simulink model "saturn_ib_stack"  (Simulink 6.2)
settings: Solver=ode4  SolverMode=SingleTasking  StartTime=0.0  StopTime=inf  FixedStep=0.005  RelTol=1e-3
values from neighbouring files (symbols this model uses):
  A_z_deg = 82.8200    (= 82.82)    [AS205_presettings.m]
  BN_1_sec = 14.4    [AS205_presettings.m]
  DeltaV_b_mps = 7.2381    [AS205_presettings.m]
  epsilon_2_sec = 15.0    (= 15)    [AS205_presettings.m]
  epsilon_prime_sec = 3.0    (= 3)    [AS205_presettings.m]
  i_deg = 28.89597    [AS205_presettings.m]
  lambda_0_deg = 102.32900    (= 102.329)    [AS205_presettings.m]
  lambda_L_deg = -80.561141    [AS205_presettings.m]
  pad_roll_L_deg = 100.0    (= 100)    [AS205_presettings.m]
  phi_L_deg = 28.521963    [AS205_presettings.m]
  phi_L_prime_deg = 28.360795    [AS205_presettings.m]
  R_L_m = 6373385.0    (= 6373385)    [AS205_presettings.m]
  R_T_m = 6570774.0    (= 6570774)    [AS205_presettings.m]
  T3_FM_sec = 6.08    [AS205_presettings.m]
  T_HSL_sec = 5.0    (= 5)    [AS205_presettings.m]
  Theta_T_deg = 0.000    (= 0)    [AS205_presettings.m]
  V_T_mps = 7780.976    [AS205_presettings.m]
  Xdotdot_VGT_mps2 = -9.251    [AS205_presettings.m]
undefined symbols (not defined in the file or in its folder): e0_0, e1_0, e2_0, e3_0, m, s
libraries: simulink x98, aerolibconvert x83, aerolibutil x63, aerolibtransform2 x34, aerolibasang x2, aerolibatmos2 x2, aerolib6dofsys x2
(part 6 of 7)

== system saturn_ib_stack/Saturn_IB_Stack/Saturn Instrument Unit (IU)/LVDA / LVDC/T4 Timer ==
  bStart : Inport  Port=1  DataType=boolean  LatchInput=off
  Clock : Clock
      settings: Decimation=10
  Constant : Constant  Value=0.0
  Data Store Memory : DataStoreMemory  DataStoreName=A  InitialValue=-1  DataType=double
  Data Store Read : DataStoreRead  DataStoreName=A  SampleTime=0
  Sum : Sum  Inputs=|+-
  Switch : Switch  Threshold=0.0
  Timer Initialization : Subsystem  TreatAsAtomicUnit=on
  T_elapsed_sec : Outport
  wires:
  bStart/1 -> Timer Initialization/Trigger
  Clock/1 -> Timer Initialization/1(In1), Sum/1
  Switch/1 -> T_elapsed_sec/1
  Sum/1 -> Switch/1
  Data Store Read/1 -> Sum/2, Switch/2
  Constant/1 -> Switch/3

== system saturn_ib_stack/Saturn_IB_Stack/Saturn Instrument Unit (IU)/ST-124M Stabilized Platform/Platform Gimbal Angles ==
  DCM : Inport  Port=1  LatchInput=off
  -sin(theta_x)cos(theta_z) : Fcn  Expr=-u(8)
  -sin(theta_y)cos(theta_z) : Fcn  Expr=-u(3)
  Mux2 : Mux  Inputs=3
  "Reshape 3x3 -> 9x1" : simulink/Math Operations/Reshape  OutputDimensionality=Customize  OutputDimensions=[9, 1]
  Trigonometric Function1 : Trigonometry  Operator=atan2
  Trigonometric Function3 : Trigonometry  Operator=atan2
  Trigonometric Function4 : Trigonometry  Operator=asin
  cos(theta_x)cos(theta_z) : Fcn  Expr=u(5)
  cos(theta_y)cos(theta_z) : Fcn  Expr=u(1)
  "sin(theta_z) " : Fcn  Expr=u(2)
  ST-124 Gimbal : Outport  InitialOutput=0
  wires:
  DCM/1 -> "Reshape 3x3 -> 9x1"/1
  "Reshape 3x3 -> 9x1"/1 -> -sin(theta_x)cos(theta_z)/1, cos(theta_x)cos(theta_z)/1, -sin(theta_y)cos(theta_z)/1, cos(theta_y)cos(theta_z)/1, "sin(theta_z) "/1
  -sin(theta_x)cos(theta_z)/1 -> Trigonometric Function1/1
  cos(theta_x)cos(theta_z)/1 -> Trigonometric Function1/2
  -sin(theta_y)cos(theta_z)/1 -> Trigonometric Function3/1
  cos(theta_y)cos(theta_z)/1 -> Trigonometric Function3/2
  Mux2/1 -> ST-124 Gimbal/1
  "sin(theta_z) "/1 -> Trigonometric Function4/1
  Trigonometric Function4/1 -> Mux2/3  "theta_z"
  Trigonometric Function1/1 -> Mux2/1  "theta_x"
  Trigonometric Function3/1 -> Mux2/2  "theta_y"

== system saturn_ib_stack/Saturn_IB_Stack/Initial Conditions/MES Transform/MES Transform/E-Frame to s-Frame (MES matrix) ==
  note: u(1)  sin Az
      | u(2)  sin Phi_L
      | u(3)  sin Theta_E
      | u(4)  cos Az
      | u(5)  cos Phi_L
      | u(6)  cos Theta_E
  note: Eqn 2.3.10
  Az phi_L Theta_E : Inport  Port=1  LatchInput=off
  11 : Fcn  Expr=u(5)*u(6)
  12 : Fcn  Expr=u(5)*u(3)
  13 : Fcn  Expr=u(2)
  21 : Fcn  Expr=u(2)*u(1)*u(6)-u(4)*u(3)
  22 : Fcn  Expr=u(2)*u(1)*u(3)+u(4)*u(6)
  23 : Fcn  Expr=-u(5)*u(1)
  31 : Fcn  Expr=-u(2)*u(4)*u(6)-u(1)*u(3)
  32 : Fcn  Expr=-u(2)*u(4)*u(3)+u(1)*u(6)
  33 : Fcn  Expr=u(5)*u(4)
  Mux : Mux  Inputs=2
  Mux2 : Mux  Inputs=9
  Reshape 9x1->3x3 : simulink/Math Operations/Reshape  OutputDimensionality=Customize  OutputDimensions=[3,3]
  SinCos3 : aerolibutil/SinCos
  DCM : Outport  InitialOutput=0
  wires:
  33/1 -> Mux2/9
  22/1 -> Mux2/5
  11/1 -> Mux2/1
  Mux2/1 -> Reshape 9x1->3x3/1
  Reshape 9x1->3x3/1 -> DCM/1
  Mux/1 -> 22/1, 11/1, 21/1, 31/1, 12/1, 32/1, 13/1, 33/1, 23/1
  23/1 -> Mux2/8
  13/1 -> Mux2/7
  32/1 -> Mux2/6
  12/1 -> Mux2/4
  31/1 -> Mux2/3
  21/1 -> Mux2/2
  Az phi_L Theta_E/1 -> SinCos3/1
  SinCos3/1 -> Mux/1
  SinCos3/2 -> Mux/2

== system saturn_ib_stack/Saturn_IB_Stack/On Pad/Initial Conditions/L/V Inertial Orientation/E-Frame to s-Frame (MES matrix) ==
  note: u(1)  sin Az
      | u(2)  sin Phi_L
      | u(3)  sin Theta_E
      | u(4)  cos Az
      | u(5)  cos Phi_L
      | u(6)  cos Theta_E
  note: Eqn 2.3.10
  Az phi_L Theta_E : Inport  Port=1  LatchInput=off
  11 : Fcn  Expr=u(5)*u(6)
  12 : Fcn  Expr=u(5)*u(3)
  13 : Fcn  Expr=u(2)
  21 : Fcn  Expr=u(2)*u(1)*u(6)-u(4)*u(3)
  22 : Fcn  Expr=u(2)*u(1)*u(3)+u(4)*u(6)
  23 : Fcn  Expr=-u(5)*u(1)
  31 : Fcn  Expr=-u(2)*u(4)*u(6)-u(1)*u(3)
  32 : Fcn  Expr=-u(2)*u(4)*u(3)+u(1)*u(6)
  33 : Fcn  Expr=u(5)*u(4)
  Mux : Mux  Inputs=2
  Mux2 : Mux  Inputs=9
  Reshape 9x1->3x3 : simulink/Math Operations/Reshape  OutputDimensionality=Customize  OutputDimensions=[3,3]
  SinCos3 : aerolibutil/SinCos
  DCM : Outport  InitialOutput=0
  wires:
  33/1 -> Mux2/9
  22/1 -> Mux2/5
  11/1 -> Mux2/1
  Mux2/1 -> Reshape 9x1->3x3/1
  Reshape 9x1->3x3/1 -> DCM/1
  Mux/1 -> 22/1, 11/1, 21/1, 31/1, 12/1, 32/1, 13/1, 33/1, 23/1
  23/1 -> Mux2/8
  13/1 -> Mux2/7
  32/1 -> Mux2/6
  12/1 -> Mux2/4
  31/1 -> Mux2/3
  21/1 -> Mux2/2
  Az phi_L Theta_E/1 -> SinCos3/1
  SinCos3/1 -> Mux/1
  SinCos3/2 -> Mux/2

== system saturn_ib_stack/Saturn_IB_Stack/On Pad/Initial Conditions/MES Transform/MES Transform ==
  A_z_deg : Inport  Port=1  LatchInput=off
  phi_L_deg : Inport  Port=2  LatchInput=off
  Theta_E_deg : Inport  Port=3  LatchInput=off
  Angle Conversion2 : aerolibconvert/Angle Conversion  IU=deg  OU=rad
  E-Frame to s-Frame (MES matrix) : Subsystem  AncestorBlock="aerolibtransform2/Euler Angles to  Direction Cosine Matrix"
      mask Type: Euler2DCM
      mask Description: Determine the 3-by-3 direction cosine matrix (DCM) transforming the E-frame to the S-Frame
      mask Display: disp('MES')
  Mux : Mux  Inputs=3
  DCM : Outport
  wires:
  phi_L_deg/1 -> Mux/2
  Theta_E_deg/1 -> Mux/3
  A_z_deg/1 -> Mux/1
  Mux/1 -> Angle Conversion2/1
  E-Frame to s-Frame (MES matrix)/1(DCM) -> DCM/1
  Angle Conversion2/1 -> E-Frame to s-Frame (MES matrix)/1(Az phi_L Theta_E)

== system saturn_ib_stack/Saturn_IB_Stack/S-IB Stage/Custom Variable Mass 6DoF (Quaternion)/Calculate DCM & Euler Angles/qdot ==
  p q r : Inport  Port=1  LatchInput=off
  q0 q1 q2 q3 : Inport  Port=2  LatchInput=off
  Constant : Constant
  Dot Product : simulink/Math Operations/Dot Product  OutDataType=sfix(16)  OutScaling=2^-10  DoSatur=off
  High Gain Quaternion Normalization : Gain  Gain=k_quat  SaturateOnIntegerOverflow=on
  Mux1 : Mux  Inputs=[3 4 1]
  Mux2 : Mux
  Sum : Sum  Inputs=|+-  SaturateOnIntegerOverflow=on  InputSameDT=on
  q0dot : Fcn  Expr=-0.5 * ( u[5]*u[1]+u[6]*u[2]+u[7]*u[3] ) + u[8]*u[4]
  q1dot : Fcn  Expr=0.5 * ( u[4]*u[1]+u[6]*u[3]-u[7]*u[2] ) + u[8]*u[5]
  q2dot : Fcn  Expr=0.5 * ( u[4]*u[2]+u[7]*u[1]-u[5]*u[3] ) + u[8]*u[6]
  q3dot : Fcn  Expr=0.5 * ( u[4]*u[3]+u[5]*u[2]-u[6]*u[1] ) + u[8]*u[7]
  qdot : Outport  InitialOutput=0
  wires:
  p q r/1 -> Mux1/1
  Dot Product/1 -> Sum/2
  High Gain Quaternion Normalization/1 -> Mux1/3
  Sum/1 -> High Gain Quaternion Normalization/1
  Constant/1 -> Sum/1
  Mux2/1 -> qdot/1
  q0dot/1 -> Mux2/1
  q1dot/1 -> Mux2/2
  q2dot/1 -> Mux2/3
  Mux1/1 -> q2dot/1, q3dot/1, q0dot/1, q1dot/1
  q3dot/1 -> Mux2/4
  q0 q1 q2 q3/1 -> Dot Product/1, Dot Product/2, Mux1/2

== system saturn_ib_stack/Saturn_IB_Stack/S-IB Stage/Custom Variable Mass 6DoF (Quaternion)/Calculate omega_dot/I x w ==
  p q r : Inport  Port=1  LatchInput=off
  Inertia : Inport  Port=2  LatchInput=off
  Product : Product  Multiplication=Matrix(*)  SaturateOnIntegerOverflow=on  InputSameDT=on
  I * w : Outport
  wires:
  p q r/1 -> Product/2
  Inertia/1 -> Product/1
  Product/1 -> I * w/1

== system saturn_ib_stack/Saturn_IB_Stack/S-IB Stage/Custom Variable Mass 6DoF (Quaternion)/Calculate omega_dot/I x w1 ==
  I_dot : Inport  Port=1  LatchInput=off
  p q r : Inport  Port=2  LatchInput=off
  Product : Product  Multiplication=Matrix(*)  SaturateOnIntegerOverflow=on  InputSameDT=on
  Id * w : Outport
  wires:
  Product/1 -> Id * w/1
  I_dot/1 -> Product/1
  p q r/1 -> Product/2

== system saturn_ib_stack/Saturn_IB_Stack/S-IB Stage/H-1 Engine Cluster/Engine 1/Triggered Timer ==
  bStart : Inport  Port=1  DataType=boolean  LatchInput=off
  Clock : Clock
      settings: Decimation=10
  Constant : Constant  Value=0.0
  Data Store Memory : DataStoreMemory  DataStoreName=A  InitialValue=-1  DataType=double
  Data Store Read : DataStoreRead  DataStoreName=A  SampleTime=0
  Sum : Sum  Inputs=|+-
  Switch : Switch  Threshold=0.0
  Timer Initialization : Subsystem  TreatAsAtomicUnit=on
  T_elapsed_sec : Outport
  wires:
  bStart/1 -> Timer Initialization/Trigger
  Clock/1 -> Timer Initialization/1(In1), Sum/1
  Switch/1 -> T_elapsed_sec/1
  Sum/1 -> Switch/1
  Data Store Read/1 -> Sum/2, Switch/2
  Constant/1 -> Switch/3

== system saturn_ib_stack/Saturn_IB_Stack/S-IB Stage/H-1 Engine Cluster/Engine 2/Triggered Timer ==
  bStart : Inport  Port=1  DataType=boolean  LatchInput=off
  Clock : Clock
      settings: Decimation=10
  Constant : Constant  Value=0.0
  Data Store Memory : DataStoreMemory  DataStoreName=A  InitialValue=-1  DataType=double
  Data Store Read : DataStoreRead  DataStoreName=A  SampleTime=0
  Sum : Sum  Inputs=|+-
  Switch : Switch  Threshold=0.0
  Timer Initialization : Subsystem  TreatAsAtomicUnit=on
  T_elapsed_sec : Outport
  wires:
  bStart/1 -> Timer Initialization/Trigger
  Clock/1 -> Timer Initialization/1(In1), Sum/1
  Switch/1 -> T_elapsed_sec/1
  Sum/1 -> Switch/1
  Data Store Read/1 -> Sum/2, Switch/2
  Constant/1 -> Switch/3

== system saturn_ib_stack/Saturn_IB_Stack/S-IB Stage/H-1 Engine Cluster/Engine 3/Triggered Timer ==
  bStart : Inport  Port=1  DataType=boolean  LatchInput=off
  Clock : Clock
      settings: Decimation=10
  Constant : Constant  Value=0.0
  Data Store Memory : DataStoreMemory  DataStoreName=A  InitialValue=-1  DataType=double
  Data Store Read : DataStoreRead  DataStoreName=A  SampleTime=0
  Sum : Sum  Inputs=|+-
  Switch : Switch  Threshold=0.0
  Timer Initialization : Subsystem  TreatAsAtomicUnit=on
  T_elapsed_sec : Outport
  wires:
  bStart/1 -> Timer Initialization/Trigger
  Clock/1 -> Timer Initialization/1(In1), Sum/1
  Switch/1 -> T_elapsed_sec/1
  Sum/1 -> Switch/1
  Data Store Read/1 -> Sum/2, Switch/2
  Constant/1 -> Switch/3

== system saturn_ib_stack/Saturn_IB_Stack/S-IB Stage/H-1 Engine Cluster/Engine 4/Triggered Timer ==
  bStart : Inport  Port=1  DataType=boolean  LatchInput=off
  Clock : Clock
      settings: Decimation=10
  Constant : Constant  Value=0.0
  Data Store Memory : DataStoreMemory  DataStoreName=A  InitialValue=-1  DataType=double
  Data Store Read : DataStoreRead  DataStoreName=A  SampleTime=0
  Sum : Sum  Inputs=|+-
  Switch : Switch  Threshold=0.0
  Timer Initialization : Subsystem  TreatAsAtomicUnit=on
  T_elapsed_sec : Outport
  wires:
  bStart/1 -> Timer Initialization/Trigger
  Clock/1 -> Timer Initialization/1(In1), Sum/1
  Switch/1 -> T_elapsed_sec/1
  Sum/1 -> Switch/1
  Data Store Read/1 -> Sum/2, Switch/2
  Constant/1 -> Switch/3

== system saturn_ib_stack/Saturn_IB_Stack/S-IB Stage/H-1 Engine Cluster/Engine 5/Triggered Timer ==
  bStart : Inport  Port=1  DataType=boolean  LatchInput=off
  Clock : Clock
      settings: Decimation=10
  Constant : Constant  Value=0.0
  Data Store Memory : DataStoreMemory  DataStoreName=A  InitialValue=-1  DataType=double
  Data Store Read : DataStoreRead  DataStoreName=A  SampleTime=0
  Sum : Sum  Inputs=|+-
  Switch : Switch  Threshold=0.0
  Timer Initialization : Subsystem  TreatAsAtomicUnit=on
  T_elapsed_sec : Outport
  wires:
  bStart/1 -> Timer Initialization/Trigger
  Clock/1 -> Timer Initialization/1(In1), Sum/1
  Switch/1 -> T_elapsed_sec/1
  Sum/1 -> Switch/1
  Data Store Read/1 -> Sum/2, Switch/2
  Constant/1 -> Switch/3

== system saturn_ib_stack/Saturn_IB_Stack/S-IB Stage/H-1 Engine Cluster/Engine 6/Triggered Timer ==
  bStart : Inport  Port=1  DataType=boolean  LatchInput=off
  Clock : Clock
      settings: Decimation=10
  Constant : Constant  Value=0.0
  Data Store Memory : DataStoreMemory  DataStoreName=A  InitialValue=-1  DataType=double
  Data Store Read : DataStoreRead  DataStoreName=A  SampleTime=0
  Sum : Sum  Inputs=|+-
  Switch : Switch  Threshold=0.0
  Timer Initialization : Subsystem  TreatAsAtomicUnit=on
  T_elapsed_sec : Outport
  wires:
  bStart/1 -> Timer Initialization/Trigger
  Clock/1 -> Timer Initialization/1(In1), Sum/1
  Switch/1 -> T_elapsed_sec/1
  Sum/1 -> Switch/1
  Data Store Read/1 -> Sum/2, Switch/2
  Constant/1 -> Switch/3

== system saturn_ib_stack/Saturn_IB_Stack/S-IB Stage/H-1 Engine Cluster/Engine 7/Triggered Timer ==
  bStart : Inport  Port=1  DataType=boolean  LatchInput=off
  Clock : Clock
      settings: Decimation=10
  Constant : Constant  Value=0.0
  Data Store Memory : DataStoreMemory  DataStoreName=A  InitialValue=-1  DataType=double
  Data Store Read : DataStoreRead  DataStoreName=A  SampleTime=0
  Sum : Sum  Inputs=|+-
  Switch : Switch  Threshold=0.0
  Timer Initialization : Subsystem  TreatAsAtomicUnit=on
  T_elapsed_sec : Outport
  wires:
  bStart/1 -> Timer Initialization/Trigger
  Clock/1 -> Timer Initialization/1(In1), Sum/1
  Switch/1 -> T_elapsed_sec/1
  Sum/1 -> Switch/1
  Data Store Read/1 -> Sum/2, Switch/2
  Constant/1 -> Switch/3

== system saturn_ib_stack/Saturn_IB_Stack/S-IB Stage/H-1 Engine Cluster/Engine 8/Triggered Timer ==
  bStart : Inport  Port=1  DataType=boolean  LatchInput=off
  Clock : Clock
      settings: Decimation=10
  Constant : Constant  Value=0.0
  Data Store Memory : DataStoreMemory  DataStoreName=A  InitialValue=-1  DataType=double
  Data Store Read : DataStoreRead  DataStoreName=A  SampleTime=0
  Sum : Sum  Inputs=|+-
  Switch : Switch  Threshold=0.0
  Timer Initialization : Subsystem  TreatAsAtomicUnit=on
  T_elapsed_sec : Outport
  wires:
  bStart/1 -> Timer Initialization/Trigger
  Clock/1 -> Timer Initialization/1(In1), Sum/1
  Switch/1 -> T_elapsed_sec/1
  Sum/1 -> Switch/1
  Data Store Read/1 -> Sum/2, Switch/2
  Constant/1 -> Switch/3

== system saturn_ib_stack/Saturn_IB_Stack/S-IB Stage/Retrorocket Motors/Time Since Engine Start/Timer Initialization ==
  In1 : Inport  Port=1  LatchInput=off
  Trigger : TriggerPort
  Data Store Write : DataStoreWrite  DataStoreName=A  SampleTime=-1
  wires:
  In1/1 -> Data Store Write/1

== system saturn_ib_stack/Saturn_IB_Stack/S-IVB Stage/Custom Variable Mass 6DoF (Quaternion)/Calculate DCM & Euler Angles/qdot ==
  p q r : Inport  Port=1  LatchInput=off
  q0 q1 q2 q3 : Inport  Port=2  LatchInput=off
  Constant : Constant
  Dot Product : simulink/Math Operations/Dot Product  OutDataType=sfix(16)  OutScaling=2^-10  DoSatur=off
  High Gain Quaternion Normalization : Gain  Gain=k_quat  SaturateOnIntegerOverflow=on
  Mux1 : Mux  Inputs=[3 4 1]
  Mux2 : Mux
  Sum : Sum  Inputs=|+-  SaturateOnIntegerOverflow=on  InputSameDT=on
  q0dot : Fcn  Expr=-0.5 * ( u[5]*u[1]+u[6]*u[2]+u[7]*u[3] ) + u[8]*u[4]
  q1dot : Fcn  Expr=0.5 * ( u[4]*u[1]+u[6]*u[3]-u[7]*u[2] ) + u[8]*u[5]
  q2dot : Fcn  Expr=0.5 * ( u[4]*u[2]+u[7]*u[1]-u[5]*u[3] ) + u[8]*u[6]
  q3dot : Fcn  Expr=0.5 * ( u[4]*u[3]+u[5]*u[2]-u[6]*u[1] ) + u[8]*u[7]
  qdot : Outport  InitialOutput=0
  wires:
  p q r/1 -> Mux1/1
  Dot Product/1 -> Sum/2
  High Gain Quaternion Normalization/1 -> Mux1/3
  Sum/1 -> High Gain Quaternion Normalization/1
  Constant/1 -> Sum/1
  Mux2/1 -> qdot/1
  q0dot/1 -> Mux2/1
  q1dot/1 -> Mux2/2
  q2dot/1 -> Mux2/3
  Mux1/1 -> q2dot/1, q3dot/1, q0dot/1, q1dot/1
  q3dot/1 -> Mux2/4
  q0 q1 q2 q3/1 -> Dot Product/1, Dot Product/2, Mux1/2

== system saturn_ib_stack/Saturn_IB_Stack/S-IVB Stage/Custom Variable Mass 6DoF (Quaternion)/Calculate omega_dot/I x w ==
  p q r : Inport  Port=1  LatchInput=off
  Inertia : Inport  Port=2  LatchInput=off
  Product : Product  Multiplication=Matrix(*)  SaturateOnIntegerOverflow=on  InputSameDT=on
  I * w : Outport
  wires:
  p q r/1 -> Product/2
  Inertia/1 -> Product/1
  Product/1 -> I * w/1

== system saturn_ib_stack/Saturn_IB_Stack/S-IVB Stage/Custom Variable Mass 6DoF (Quaternion)/Calculate omega_dot/I x w1 ==
  I_dot : Inport  Port=1  LatchInput=off
  p q r : Inport  Port=2  LatchInput=off
  Product : Product  Multiplication=Matrix(*)  SaturateOnIntegerOverflow=on  InputSameDT=on
  Id * w : Outport
  wires:
  Product/1 -> Id * w/1
  I_dot/1 -> Product/1
  p q r/1 -> Product/2

== system saturn_ib_stack/Saturn_IB_Stack/S-IVB Stage/J-2 Engine/Thrust Model/Time Since Engine Start ==
  bStart : Inport  Port=1  DataType=boolean  LatchInput=off
  Clock : Clock
      settings: Decimation=10
  Constant : Constant  Value=0.0
  Data Store Memory : DataStoreMemory  DataStoreName=A  InitialValue=-1  DataType=double
  Data Store Read : DataStoreRead  DataStoreName=A  SampleTime=0
  Sum : Sum  Inputs=|+-
  Switch : Switch  Threshold=0.0
  Timer Initialization : Subsystem  TreatAsAtomicUnit=on
  T_elapsed_sec : Outport
  wires:
  bStart/1 -> Timer Initialization/Trigger
  Clock/1 -> Timer Initialization/1(In1), Sum/1
  Switch/1 -> T_elapsed_sec/1
  Sum/1 -> Switch/1
  Data Store Read/1 -> Sum/2, Switch/2
  Constant/1 -> Switch/3

== system saturn_ib_stack/Saturn_IB_Stack/S-IVB Stage/J-2 Engine/Thrust Model/Time Since Shutdown ==
  bStart : Inport  Port=1  DataType=boolean  LatchInput=off
  Clock : Clock
      settings: Decimation=10
  Constant : Constant  Value=0.0
  Data Store Memory : DataStoreMemory  DataStoreName=A  InitialValue=-1  DataType=double
  Data Store Read : DataStoreRead  DataStoreName=A  SampleTime=0
  Sum : Sum  Inputs=|+-
  Switch : Switch  Threshold=0.0
  Timer Initialization : Subsystem  TreatAsAtomicUnit=on
  T_elapsed_sec : Outport
  wires:
  bStart/1 -> Timer Initialization/Trigger
  Clock/1 -> Timer Initialization/1(In1), Sum/1
  Switch/1 -> T_elapsed_sec/1
  Sum/1 -> Switch/1
  Data Store Read/1 -> Sum/2, Switch/2
  Constant/1 -> Switch/3

== system saturn_ib_stack/Saturn_IB_Stack/S-IVB Stage/Ullage Rocket Motors/Time Since Engine Start/Timer Initialization ==
  In1 : Inport  Port=1  LatchInput=off
  Trigger : TriggerPort
  Data Store Write : DataStoreWrite  DataStoreName=A  SampleTime=-1
  wires:
  In1/1 -> Data Store Write/1

== system saturn_ib_stack/Saturn_IB_Stack/Saturn Instrument Unit (IU)/Flight Control Computer/S-IVB Stage Timer/Timer Initialization ==
  In1 : Inport  Port=1  LatchInput=off
  Trigger : TriggerPort
  Data Store Write : DataStoreWrite  DataStoreName=A  SampleTime=-1
  wires:
  In1/1 -> Data Store Write/1

== system saturn_ib_stack/Saturn_IB_Stack/Saturn Instrument Unit (IU)/Flight Control Computer/Spatial Attitude Control System/Derived Rate Modulator ==
  In : Inport  Port=1  LatchInput=off
  +Uoff +Uon : Relay  OnSwitchValue=1.0  OffSwitchValue=0.9524
  -Uoff -Uon : Relay  OnSwitchValue=1.0  OffSwitchValue=0.9524  OnOutputValue=-1
  Compare To Zero : simulink/Logic and Bit Operations/Compare To Zero  relop=<  LogicOutDataTypeMode=boolean  ZeroCross=off
  Compare To Zero1 : simulink/Logic and Bit Operations/Compare To Zero  relop=>  LogicOutDataTypeMode=boolean  ZeroCross=off
  Sum : Sum  Inputs=|+-
  Sum5 : Sum  Inputs=+|+
  Transfer Fcn : TransferFcn  Orientation=left  Numerator=[0.476]  Denominator=[0.65 1]
  Unary Minus : simulink/Math Operations/Unary Minus  DoSatur=off
  A : Outport
  B : Outport  Port=2
  wires:
  Transfer Fcn/1 -> Sum/2
  -Uoff -Uon/1 -> Sum5/2
  +Uoff +Uon/1 -> Sum5/1
  Unary Minus/1 -> -Uoff -Uon/1
  Sum/1 -> +Uoff +Uon/1, Unary Minus/1
  Sum5/1 -> Compare To Zero1/1, Compare To Zero/1, Transfer Fcn/1
  In/1 -> Sum/1
  Compare To Zero1/1 -> A/1
  Compare To Zero/1 -> B/1

== system saturn_ib_stack/Saturn_IB_Stack/Saturn Instrument Unit (IU)/Flight Control Computer/Spatial Attitude Control System/Derived Rate Modulator (Pitch) ==
  In : Inport  Port=1  LatchInput=off
  +Uoff +Uon : Relay  OnSwitchValue=1.0  OffSwitchValue=0.9524
  -Uoff -Uon : Relay  OnSwitchValue=1.0  OffSwitchValue=0.9524  OnOutputValue=-1
  Compare To Zero : simulink/Logic and Bit Operations/Compare To Zero  relop=<  LogicOutDataTypeMode=boolean  ZeroCross=off
  Compare To Zero1 : simulink/Logic and Bit Operations/Compare To Zero  relop=>  LogicOutDataTypeMode=boolean  ZeroCross=off
  Sum : Sum  Inputs=|+-
  Sum5 : Sum  Inputs=+|+
  Transfer Fcn : TransferFcn  Orientation=left  Numerator=[0.476]  Denominator=[0.65 1]
  Unary Minus : simulink/Math Operations/Unary Minus  DoSatur=off
  A : Outport
  B : Outport  Port=2
  wires:
  Transfer Fcn/1 -> Sum/2
  -Uoff -Uon/1 -> Sum5/2
  +Uoff +Uon/1 -> Sum5/1
  Unary Minus/1 -> -Uoff -Uon/1
  Sum/1 -> +Uoff +Uon/1, Unary Minus/1
  Sum5/1 -> Transfer Fcn/1, Compare To Zero1/1, Compare To Zero/1
  In/1 -> Sum/1
  Compare To Zero1/1 -> A/1
  Compare To Zero/1 -> B/1

== system saturn_ib_stack/Saturn_IB_Stack/Saturn Instrument Unit (IU)/Flight Control Computer/Spatial Attitude Control System/Derived Rate Modulator1 ==
  In : Inport  Port=1  LatchInput=off
  +Uoff +Uon : Relay  OnSwitchValue=1.0  OffSwitchValue=0.9524
  -Uoff -Uon : Relay  OnSwitchValue=1.0  OffSwitchValue=0.9524  OnOutputValue=-1
  Compare To Zero : simulink/Logic and Bit Operations/Compare To Zero  relop=<  LogicOutDataTypeMode=boolean  ZeroCross=off
  Compare To Zero1 : simulink/Logic and Bit Operations/Compare To Zero  relop=>  LogicOutDataTypeMode=boolean  ZeroCross=off
  Sum : Sum  Inputs=|+-
  Sum5 : Sum  Inputs=+|+
  Transfer Fcn : TransferFcn  Orientation=left  Numerator=[0.476]  Denominator=[0.65 1]
  Unary Minus : simulink/Math Operations/Unary Minus  DoSatur=off
  A : Outport
  B : Outport  Port=2
  wires:
  Transfer Fcn/1 -> Sum/2
  -Uoff -Uon/1 -> Sum5/2
  +Uoff +Uon/1 -> Sum5/1
  Unary Minus/1 -> -Uoff -Uon/1
  Sum/1 -> +Uoff +Uon/1, Unary Minus/1
  Sum5/1 -> Compare To Zero1/1, Compare To Zero/1, Transfer Fcn/1
  In/1 -> Sum/1
  Compare To Zero1/1 -> A/1
  Compare To Zero/1 -> B/1

== system saturn_ib_stack/Saturn_IB_Stack/Saturn Instrument Unit (IU)/LVDA / LVDC/LVDC Chi command angles (Time Tilt)/Rate Limiter Dynamic ==
  up : Inport  Port=1  LatchInput=off
  u : Inport  Port=2  LatchInput=off
  lo : Inport  Port=3  LatchInput=off
  Delay Input2 : UnitDelay  Description=Store in Global RAM  Orientation=left  X0="[-17.18  0.0 0.0]"  SampleTime=-1
  Difference Inputs1 : Sum  Description=Add in CPU  Inputs=+-  OutDataType=uint(8)  OutScaling=1
  Difference Inputs2 : Sum  Description=Add in CPU  OutDataType=uint(8)  OutScaling=1
  FixPt Data Type Duplicate : simulink/Signal Attributes/Data Type Duplicate  NumInputPorts=7
  Saturation Dynamic : simulink/Discontinuities/Saturation Dynamic
  delta fall limit : Product  Inputs=**  OutDataType=uint(16)  OutScaling=2^-10  SaturateOnIntegerOverflow=on
  delta rise limit : Product  Inputs=**  OutDataType=uint(16)  OutScaling=2^-10  SaturateOnIntegerOverflow=on
  sample time : simulink/Math Operations/Weighted Sample Time Math  TsampMathOp=Ts Only  weightValue=1  TsampMathImp=Online Calculations  DoSatur=off
  Y : Outport  PortDimensions=3  InitialOutput=0
  wires:
  Difference Inputs1/1 -> FixPt Data Type Duplicate/4, Saturation Dynamic/2  "( U(k) - Y(k-1) )"
  u/1 -> Difference Inputs1/1, FixPt Data Type Duplicate/5, sample time/1  "U(k)"
  delta fall limit/1 -> FixPt Data Type Duplicate/3, Saturation Dynamic/3
  Saturation Dynamic/1 -> Difference Inputs2/1, FixPt Data Type Duplicate/7
  Delay Input2/1 -> Difference Inputs2/2, Difference Inputs1/2, FixPt Data Type Duplicate/2  "Y(k-1)"
  Difference Inputs2/1 -> Y/1, Delay Input2/1, FixPt Data Type Duplicate/1  "Y(k)"
  up/1 -> delta rise limit/1
  delta rise limit/1 -> FixPt Data Type Duplicate/6, Saturation Dynamic/1
  lo/1 -> delta fall limit/1
  sample time/1 -> delta fall limit/2, delta rise limit/2

== system saturn_ib_stack/Saturn_IB_Stack/Saturn Instrument Unit (IU)/LVDA / LVDC/LVDC Chi command angles (Time Tilt)/Store Chi Command Angles ==
  In1 : Inport  Port=1  LatchInput=off
  Enable : EnablePort
  Data Store Write : DataStoreWrite  DataStoreName=Chi_X_deg  SampleTime=-1
  Data Store Write1 : DataStoreWrite  DataStoreName=Chi_Y_deg  SampleTime=-1
  Data Store Write2 : DataStoreWrite  DataStoreName=Chi_Z_deg  SampleTime=-1
  Demux : Demux  Outputs=3
  wires:
  Demux/1 -> Data Store Write/1
  Demux/3 -> Data Store Write2/1
  Demux/2 -> Data Store Write1/1
  In1/1 -> Demux/1

== system saturn_ib_stack/Saturn_IB_Stack/Saturn Instrument Unit (IU)/LVDA / LVDC/LVDC Iterative Guidance Mode/DeltaT_b ==
  V_mps : Inport  Port=1  LatchInput=off
  V_prime_mps : Inport  Port=2  LatchInput=off
  Enable : EnablePort
  Constant : Constant  Value=delta_T_sec
  Constant1 : Constant  Value=DeltaV_b_mps
  Data Store Write : DataStoreWrite  DataStoreName=DeltaT_b_sec  SampleTime=-1
  Divide : Product  Inputs=**/  OutScaling=2^-10
  Sum : Sum  Inputs=|+-
  wires:
  V_mps/1 -> Sum/1
  V_prime_mps/1 -> Sum/2
  Constant1/1 -> Divide/1
  Constant/1 -> Divide/2
  Sum/1 -> Divide/3
  Divide/1 -> Data Store Write/1

== system saturn_ib_stack/Saturn_IB_Stack/Saturn Instrument Unit (IU)/LVDA / LVDC/LVDC Iterative Guidance Mode/Estimated Velocity-to-be-gained ==
  note: Eqn. 4.4.46
  note: Eqn. 4.4.47
  V_TV_bar : Inport  Port=1  LatchInput=off
  V_V_bar : Inport  Port=2  LatchInput=off
  G_TV_bar : Inport  Port=3  LatchInput=off
  G_V_bar : Inport  Port=4  LatchInput=off
  T_star : Inport  Port=5  LatchInput=off
  Add8 : Sum  OutScaling=2^-10
  Add9 : Sum  Inputs=+--  OutScaling=2^-10
  Gain : Gain  Gain=0.5
  Product12 : Product  RndMeth=Zero
  Delta_V_prime_V_bar : Outport
  G_star_V_bar : Outport  Port=2
  wires:
  Add8/1 -> Gain/1
  Gain/1 -> Product12/2, G_star_V_bar/1
  T_star/1 -> Product12/1
  Product12/1 -> Add9/3
  V_TV_bar/1 -> Add9/1
  V_V_bar/1 -> Add9/2
  Add9/1 -> Delta_V_prime_V_bar/1
  G_TV_bar/1 -> Add8/1
  G_V_bar/1 -> Add8/2

== system saturn_ib_stack/Saturn_IB_Stack/Saturn Instrument Unit (IU)/LVDA / LVDC/LVDC Iterative Guidance Mode/HSL Cutoff Timing ==
  note: Cutoff is described in EDD section 4.4.2.4.
      | This doesn't quite implement the sequence descibed in that section, but
      | it is awfully close
  Enable : EnablePort
  Compare To Constant : simulink/Logic and Bit Operations/Compare To Constant  relop=<=  const=0.04  LogicOutDataTypeMode=boolean  ZeroCross=off
  Compare To Constant1 : simulink/Logic and Bit Operations/Compare To Constant  relop===  const=1  LogicOutDataTypeMode=uint8  ZeroCross=off
  Constant : Constant  Value=0.04
  Constant1 : Constant  Value=2  OutDataTypeMode=int32  SampleTime=0.04
  Data Store Read : DataStoreRead  DataStoreName=T_3_i_sec  SampleTime=0.04
  Data Store Read1 : DataStoreRead  DataStoreName=nHSLActive  SampleTime=0.04
  Data Store Read2 : DataStoreRead  DataStoreName=DeltaT_b_sec  SampleTime=0.04
  Data Store Write : DataStoreWrite  DataStoreName=T_3_i_sec  SampleTime=-1
  Data Store Write1 : DataStoreWrite  DataStoreName=nHSLActive  SampleTime=-1
  Ground : Ground
  S-Frame Solution1 : Scope  NumInputPorts=3
      settings: TimeRange=1.399999999999977  YMin=0~-1~-1  YMax=2~1~3  SaveName=ScopeData9
  Sum : Sum  Inputs=+--
  Switch : Switch  Criteria=u2 ~= 0
  bCutoff : Outport  DataType=boolean
  wires:
  Constant/1 -> Sum/2
  Sum/1 -> Data Store Write/1, Compare To Constant/1, S-Frame Solution1/1
  Data Store Read/1 -> Sum/1
  Compare To Constant/1 -> bCutoff/1
  Data Store Read1/1 -> Compare To Constant1/1, S-Frame Solution1/3
  Compare To Constant1/1 -> Switch/2
  Switch/1 -> Sum/3
  Data Store Read2/1 -> Switch/1, S-Frame Solution1/2
  Ground/1 -> Switch/3
  Constant1/1 -> Data Store Write1/1

== system saturn_ib_stack/Saturn_IB_Stack/Saturn Instrument Unit (IU)/LVDA / LVDC/LVDC Iterative Guidance Mode/IGM Chi Steering ==
  Chi_Y : Inport  Port=1  LatchInput=off
  Chi_Z : Inport  Port=2  LatchInput=off
  Enable : EnablePort
  Data Store Write3 : DataStoreWrite  DataStoreName=Chi_Y_deg  SampleTime=-1
  Data Store Write4 : DataStoreWrite  DataStoreName=Chi_Z_deg  SampleTime=-1
  wires:
  Chi_Y/1 -> Data Store Write3/1
  Chi_Z/1 -> Data Store Write4/1

== system saturn_ib_stack/Saturn_IB_Stack/Saturn Instrument Unit (IU)/LVDA / LVDC/LVDC Iterative Guidance Mode/IGM First Phase ==
  MF_S : Inport  Port=1  PortDimensions=1  DataType=double  LatchInput=off
  Action Port : ActionPort  ActionType=case
  Constant1 : Constant  Value=delta_T_sec
  Data Store Read : DataStoreRead  DataStoreName=T_1_i_sec  SampleTime=1.6
  Data Store Read1 : DataStoreRead  Priority=1  DataStoreName=tau_3_sec  SampleTime=1.6
  Data Store Read2 : DataStoreRead  Priority=1  DataStoreName=T_3_i_sec  SampleTime=1.6
  Data Store Write1 : DataStoreWrite  DataStoreName=T_1_i_sec  SampleTime=-1
  Gain2 : Gain  Gain=V_ex1_mps
  If2 : If  IfExpression=u1 <= delta_T_sec  ShowElse=off
  Mux2 : Mux
  "Set nIGMMode to \"1\"" : Subsystem  TreatAsAtomicUnit=on
  Sum4 : Sum  Inputs=|+-
  tau_values : Outport  OutputWhenDisabled=reset  InitialOutput=[0.0 0.0 0.0 0.0]
  wires:
  Constant1/1 -> Sum4/2
  Sum4/1 -> Data Store Write1/1
  Data Store Read/1 -> Sum4/1, Mux2/2, If2/1
  Gain2/1 -> Mux2/1
  MF_S/1 -> Gain2/1
  Data Store Read1/1 -> Mux2/3
  Data Store Read2/1 -> Mux2/4
  Mux2/1 -> tau_values/1
  If2/1 -> "Set nIGMMode to \"1\""/Action

== system saturn_ib_stack/Saturn_IB_Stack/Saturn Instrument Unit (IU)/LVDA / LVDC/LVDC Iterative Guidance Mode/IGM Intermediate Parameters ==
  note: eqn. 4.4.20
  note: eqn. 4.4.21
  note: eqn. 4.4.22
  note: eqn. 4.4.23
  note: eqn. 4.4.24
  note: eqn. 4.4.25
  note: eqn. 4.4.26
  note: eqn. 4.4.27
  note: eqn. 4.4.28
  note: From EDD, pages I-14-17 through I-14-18
  tau_1_sec : Inport  Port=1  LatchInput=off
  T_1_i_sec : Inport  Port=2  LatchInput=off
  tau_3_sec : Inport  Port=3  LatchInput=off
  T_3_i_sec : Inport  Port=4  LatchInput=off
  Add{,1,3..6,8} (7 alike) : Sum  Inputs=+-  OutScaling=2^-10
  Add2 : Sum  Inputs=-+  OutScaling=2^-10
  Add7 : Sum  OutScaling=2^-10
  Divide : Product  Inputs=*/  OutScaling=2^-10
  Divide{1..5,7} (6 alike) : Product  Inputs=**  OutScaling=2^-10
  Divide6 : Product  Inputs=*/  OutScaling=2^-10
  Gain : Gain  Gain=V_ex1_mps
  Gain1 : Gain  Gain=V_ex1_mps
  Gain2 : Gain  Gain=0.5
  Gain3 : Gain  Gain=V_ex1_mps
  Gain5 : Gain  Gain=V_ex3_mps
  Gain6 : Gain  Gain=V_ex3_mps
  Math Function : Math  Operator=log  SaturateOnIntegerOverflow=on
  Math Function1 : Math  Operator=square  SaturateOnIntegerOverflow=on
  Math Function2 : Math  Operator=log  SaturateOnIntegerOverflow=on
  Polynomial : simulink/Math Operations/Polynomial  coefs=[V_ex1_mps/6.0 0.0 0.0 0.0]
  L1 : Outport
  J1 : Outport  Port=2
  S1 : Outport  Port=3
  Q1 : Outport  Port=4
  P1 : Outport  Port=5
  U1 : Outport  Port=6
  L_prime_3 : Outport  Port=7
  L_prime_y : Outport  Port=8
  J_prime_3 : Outport  Port=9
  wires:
  Divide/1 -> Math Function/1
  Math Function/1 -> Gain/1
  Gain/1 -> Divide1/1, Divide2/1, L1/1, Add7/1
  tau_1_sec/1 -> Divide/1, Add/1, Divide1/2, Divide3/2, Divide4/2, Divide5/2
  T_1_i_sec/1 -> Add/2, Gain1/1, Divide2/2, Math Function1/1, Polynomial/1
  Add/1 -> Divide/2
  Gain1/1 -> Add1/2
  Divide1/1 -> Add1/1
  Add1/1 -> Add2/1, J1/1, Divide4/1
  Divide2/1 -> Add2/2
  Add2/1 -> S1/1, Divide3/1
  Math Function1/1 -> Gain3/1
  Gain3/1 -> Gain2/1
  Gain2/1 -> Add3/2, Add4/2
  Divide3/1 -> Add3/1
  Add3/1 -> Q1/1, Divide5/1
  Divide4/1 -> Add4/1
  Add4/1 -> P1/1
  Add5/1 -> U1/1
  Divide5/1 -> Add5/1
  Divide6/1 -> Math Function2/1
  tau_3_sec/1 -> Divide6/1, Add6/1, Divide7/2
  Add6/1 -> Divide6/2
  Math Function2/1 -> Gain5/1
  T_3_i_sec/1 -> Add6/2, Gain6/1
  Gain5/1 -> L_prime_3/1, Add7/2, Divide7/1
  Add7/1 -> L_prime_y/1
  Add8/1 -> J_prime_3/1
  Gain6/1 -> Add8/2
  Divide7/1 -> Add8/1
  Polynomial/1 -> Add5/2

== system saturn_ib_stack/Saturn_IB_Stack/Saturn Instrument Unit (IU)/LVDA / LVDC/LVDC Iterative Guidance Mode/IGM Phase2 (HSL first pass) ==
  note: Eqn 4.4.91 (modified)
  note: Eqn. 4.4.92
  note: Eqn. 4.4.93
  V_mps : Inport  Port=1  PortDimensions=1  DataType=double  LatchInput=off
  V_prime_mps : Inport  Port=2  PortDimensions=1  DataType=double  LatchInput=off
  V_prime_prime_mps : Inport  Port=3  PortDimensions=1  DataType=double  LatchInput=off
  Action Port : ActionPort  InitializeStates=reset  ActionType=case
  Constant1 : Constant  Value=V_T_mps
  Constant2 : Constant  Value=delta_T_sec
  Constant3 : Constant  Value=DeltaV_b_mps
  Data Store Read1 : DataStoreRead  DataStoreName=tau_1_sec  SampleTime=1.6
  Data Store Read2 : DataStoreRead  DataStoreName=T_1_i_sec  SampleTime=1.6
  Data Store Read3 : DataStoreRead  DataStoreName=tau_3_sec  SampleTime=1.6
  Data Store Read4 : DataStoreRead  DataStoreName=T_3_i_sec  SampleTime=1.6
  Data Store Read5 : DataStoreRead  DataStoreName=DeltaT_b_sec  SampleTime=1.6
  Data Store Write2 : DataStoreWrite  DataStoreName=T_3_i_sec  SampleTime=-1
  Divide : Product  Inputs=*/  OutScaling=2^-10
  Divide1 : Product  Inputs=*/  OutScaling=2^-10
  Divide2 : Product  Inputs=*/  OutScaling=2^-10
  If1 : If  NumInputs=2  IfExpression=u1 <= u2  ShowElse=off
  Mux2 : Mux
  Product{,1,3..4} (4 alike) : Product  RndMeth=Zero
  Product2 : Product  Inputs=3  RndMeth=Zero
  Set HSL Mode : Subsystem  TreatAsAtomicUnit=on
  Subtract1 : Sum  Inputs=+-  OutScaling=2^-10
  Subtract2 : Sum  Inputs=+-  OutScaling=2^-10
  Subtract3 : Sum  Inputs=+--  OutScaling=2^-10
  Subtract4 : Sum  Inputs=+-  OutScaling=2^-10
  Subtract5 : Sum  OutScaling=2^-10
  Subtract6 : Sum  OutScaling=2^-10
  Subtract7 : Sum  OutScaling=2^-10
  Sum : Sum  Inputs=|++
  T_HSL : Constant  Value=T_HSL_sec
  tau_values : Outport  OutputWhenDisabled=reset  InitialOutput=[0.0 0.0 0.0 0.0]
  wires:
  Mux2/1 -> tau_values/1
  Data Store Read1/1 -> Mux2/1
  Data Store Read2/1 -> Mux2/2
  V_mps/1 -> Subtract1/1, [V_mps]
  Data Store Read3/1 -> Mux2/3
  V_prime_mps/1 -> Subtract1/2, Subtract2/1
  V_prime_prime_mps/1 -> Subtract2/2
  Subtract1/1 -> Product/2, Divide1/1
  Subtract2/1 -> Product1/2
  Constant2/1 -> Product1/1, Product/1, Subtract5/1, Subtract5/2, Product2/2, Product2/1, Divide1/2, Product3/2
  Product/1 -> Subtract4/1
  Product1/1 -> Subtract4/2
  Subtract5/1 -> Product2/3
  Product2/1 -> Divide/2
  Subtract4/1 -> Divide/1
  Divide/1 -> Product3/1, [A_prime_prime]  "A_prime_prime"
  Product3/1 -> Subtract6/1
  Divide1/1 -> Subtract6/2
  Constant1/1 -> Subtract3/1
  Constant3/1 -> Subtract3/2
  Subtract3/1 -> Divide2/1
  Divide2/1 -> Data Store Write2/1, Mux2/4, If1/1
  Subtract6/1 -> [A_prime]
  [V_mps] -> Subtract3/3
  Data Store Read4/1 -> Product4/2
  [A_prime_prime] -> Product4/1
  [A_prime] -> Subtract7/1
  Product4/1 -> Subtract7/2
  Subtract7/1 -> Divide2/2
  If1/1 -> Set HSL Mode/Action
  Sum/1 -> If1/2
  T_HSL/1 -> Sum/1
  Data Store Read5/1 -> Sum/2

== system saturn_ib_stack/Saturn_IB_Stack/Saturn Instrument Unit (IU)/LVDA / LVDC/LVDC Iterative Guidance Mode/IGM Phase2 (artificial tau complete) ==
  note: Eqn 4.4.17
  note: Eqn 4.4.16
  MF_S : Inport  Port=1  PortDimensions=1  DataType=double  LatchInput=off
  Action Port : ActionPort  InitializeStates=reset  ActionType=case
  Constant1 : Constant  Value=delta_T_sec
  Data Store Read1 : DataStoreRead  DataStoreName=tau_1_sec  SampleTime=1.6
  Data Store Read2 : DataStoreRead  DataStoreName=T_1_i_sec  SampleTime=1.6
  Data Store Read4 : DataStoreRead  DataStoreName=T_3_i_sec  SampleTime=1.6
  Data Store Read5 : DataStoreRead  DataStoreName=DeltaT_b_sec  SampleTime=1.6
  Data Store Write1 : DataStoreWrite  DataStoreName=T_3_i_sec  SampleTime=-1
  Data Store Write5 : DataStoreWrite  DataStoreName=tau_3_sec  SampleTime=-1
  Gain1 : Gain  Gain=V_ex3_mps
  If1 : If  NumInputs=2  IfExpression=u1 <= u2  ShowElse=off
  If2 : If  NumInputs=2  IfExpression=u1 <= u2  ShowElse=off
  Mux2 : Mux
  Set HSL Mode : Subsystem  TreatAsAtomicUnit=on
  Set Terminal Steering Mode : Subsystem  TreatAsAtomicUnit=on
  Subtract3 : Sum  Inputs=+-  OutScaling=2^-10
  Sum : Sum  Inputs=|++
  T_HSL_sec : Constant  Value=T_HSL_sec
  epsilon 2 (from EDD) : Constant  Value=epsilon_2_sec
  tau_values : Outport  OutputWhenDisabled=reset  InitialOutput=[0.0 0.0 0.0 0.0]
  wires:
  Mux2/1 -> tau_values/1
  Data Store Read1/1 -> Mux2/1
  Data Store Read2/1 -> Mux2/2
  Subtract3/1 -> Data Store Write1/1, Mux2/4
  Constant1/1 -> Subtract3/2
  Gain1/1 -> Mux2/3, Data Store Write5/1
  Data Store Read4/1 -> Subtract3/1, If1/1, If2/1
  MF_S/1 -> Gain1/1
  If1/1 -> Set Terminal Steering Mode/Action
  epsilon 2 (from EDD)/1 -> If1/2
  If2/1 -> Set HSL Mode/Action
  Data Store Read5/1 -> Sum/2
  T_HSL_sec/1 -> Sum/1
  Sum/1 -> If2/2

== system saturn_ib_stack/Saturn_IB_Stack/Saturn Instrument Unit (IU)/LVDA / LVDC/LVDC Iterative Guidance Mode/IGM Phase2 (artificial tau mode) ==
  note: Eqn. 4.4.9
  note: Eqn. 4.4.10
  note: Eqn. 4.4.11
  note: Skylab EDD call this Mdot_2
  note: Eqn 4.4.12
  note: Eqn 4.4.13
  note: P_CMR??
  note: Eqn 4.4.14
  note: Eqn 4.4.15
  MF_S : Inport  Port=1  PortDimensions=1  DataType=double  LatchInput=off
  Action Port : ActionPort  InitializeStates=reset  ActionType=case
  Add : Sum  OutScaling=2^-10
  Add1 : Sum  Inputs=+-  OutScaling=2^-10
  Constant : Constant  Value=4.0
  Constant1 : Constant  Value=delta_T_sec
  Constant2 : Constant  Value=tau_1_0_sec
  Constant3 : Constant  Value=0.0
  Constant4 : Constant  Value=T10_sec
  Constant5 : Constant  Value=Mdot_1_kg_per_sec
  Constant6 : Constant  Value=C_0_sec
  Data Store Read1 : DataStoreRead  DataStoreName=P_C_sec  SampleTime=1.6
  Data Store Read3 : DataStoreRead  DataStoreName=tau_1_sec  SampleTime=1.6
  Data Store Read4 : DataStoreRead  Priority=1  DataStoreName=T_3_i_sec  SampleTime=1.6
  Data Store Write2 : DataStoreWrite  DataStoreName=T_1_i_sec  SampleTime=-1
  Data Store Write3 : DataStoreWrite  DataStoreName=alpha_f  SampleTime=-1
  Data Store Write4 : DataStoreWrite  DataStoreName=tau_3_N_sec  SampleTime=-1
  Data Store Write5 : DataStoreWrite  DataStoreName=P_C_sec  SampleTime=-1
  Data Store Write6 : DataStoreWrite  DataStoreName=tau_3_sec  SampleTime=-1
  Divide : Product  Inputs=*/  OutScaling=2^-10
  Divide1 : Product  Inputs=*/  OutScaling=2^-10
  Divide2 : Product  Inputs=***  OutScaling=2^-10
  Divide3 : Product  Inputs=*/  OutScaling=2^-10
  Gain : Gain  Gain=V_ex3_mps
  If2 : If  NumInputs=2  IfExpression=u1 >= u2  ShowElse=off
  M_GR : Constant  Value=124558.41
  M_GR1 : Constant  Value=Mdot_3_kg_per_sec
  Math Function : Math  Operator=pow  SaturateOnIntegerOverflow=on
  Mux2 : Mux
  Product : Product  RndMeth=Zero
  "Set nIGMMode to \"3\"" : Subsystem  TreatAsAtomicUnit=on
  Subtract : Sum  Inputs=+-  OutScaling=2^-10
  Subtract1 : Sum  OutScaling=2^-10
  Subtract2 : Sum  Inputs=+-  OutScaling=2^-10
  Subtract3 : Sum  OutScaling=2^-10
  Subtract4 : Sum  Inputs=+-  OutScaling=2^-10
  tau_values : Outport  PortDimensions=4  OutputWhenDisabled=reset  InitialOutput=[0.0 0.0 0.0 0.0]
  wires:
  Mux2/1 -> tau_values/1
  Divide/1 -> Data Store Write3/1, Divide2/1
  Add/1 -> Divide/2
  Data Store Read3/1 -> Add/2, Mux2/1
  Constant2/1 -> Divide/1
  Constant4/1 -> Add/1, Divide2/3
  Constant3/1 -> Data Store Write2/1, Mux2/2
  Divide1/1 -> Data Store Write4/1, Subtract/1
  M_GR1/1 -> Divide1/2
  Add1/1 -> Divide1/1
  M_GR/1 -> Add1/1
  Divide2/1 -> Add1/2
  Constant5/1 -> Divide2/2
  Gain/1 -> Subtract2/1
  Subtract/1 -> Subtract2/2, Subtract1/1
  Data Store Read1/1 -> Subtract/2, Divide3/1, Subtract3/1, If2/1
  Constant/1 -> Math Function/2
  Subtract2/1 -> Product/1
  Product/1 -> Subtract1/2
  Subtract1/1 -> Data Store Write6/1, Mux2/3
  Math Function/1 -> Product/2
  Divide3/1 -> Math Function/1
  Subtract3/1 -> Data Store Write5/1
  Constant1/1 -> Subtract3/2, Subtract4/2
  Constant6/1 -> Divide3/2, Subtract4/1
  MF_S/1 -> Gain/1
  Data Store Read4/1 -> Mux2/4
  If2/1 -> "Set nIGMMode to \"3\""/Action
  Subtract4/1 -> If2/2

== system saturn_ib_stack/Saturn_IB_Stack/Saturn Instrument Unit (IU)/LVDA / LVDC/LVDC Iterative Guidance Mode/IGM Phase2 (first BML) ==
  note: Eqn. 4.4.9
  note: Eqn. 4.4.10
  note: Eqn. 4.4.11
  note: Skylab EDD call this Mdot_2
  note: Eqn 4.4.12
  note: Eqn 4.4.13
  note: P_CMR??
  note: Eqn 4.4.14
  note: Eqn 4.4.15
  MF_S : Inport  Port=1  PortDimensions=1  DataType=double  LatchInput=off
  Action Port : ActionPort  InitializeStates=reset  ActionType=case
  Add : Sum  OutScaling=2^-10
  Add1 : Sum  Inputs=+-  OutScaling=2^-10
  Constant : Constant  Value=4.0
  Constant1 : Constant  Value=delta_T_sec
  Constant2 : Constant  Value=tau_1_0_sec
  Constant3 : Constant  Value=0.0
  Constant4 : Constant  Value=T10_sec
  Constant5 : Constant  Value=Mdot_1_kg_per_sec
  Constant6 : Constant  Value=C_0_sec
  Data Store Read1 : DataStoreRead  DataStoreName=P_C_sec  SampleTime=1.6
  Data Store Read3 : DataStoreRead  DataStoreName=tau_1_sec  SampleTime=1.6
  Data Store Read4 : DataStoreRead  Priority=1  DataStoreName=T_3_i_sec  SampleTime=1.6
  Data Store Write : DataStoreWrite  DataStoreName=nIGMMode  SampleTime=-1
  Data Store Write2 : DataStoreWrite  DataStoreName=T_1_i_sec  SampleTime=-1
  Data Store Write3 : DataStoreWrite  DataStoreName=alpha_f  SampleTime=-1
  Data Store Write4 : DataStoreWrite  DataStoreName=tau_3_N_sec  SampleTime=-1
  Data Store Write5 : DataStoreWrite  DataStoreName=P_C_sec  SampleTime=-1
  Data Store Write6 : DataStoreWrite  DataStoreName=tau_3_sec  SampleTime=-1
  Display : Display
  Divide : Product  Inputs=*/  OutScaling=2^-10
  Divide1 : Product  Inputs=*/  OutScaling=2^-10
  Divide2 : Product  Inputs=***  OutScaling=2^-10
  Divide3 : Product  Inputs=*/  OutScaling=2^-10
  Gain : Gain  Gain=V_ex3_mps
  M_GR : Constant  Value=124558.41
  M_GR1 : Constant  Value=Mdot_3_kg_per_sec
  Math Function : Math  Operator=pow  SaturateOnIntegerOverflow=on
  Mux2 : Mux
  Phase 2 : Constant  Value=2  OutDataTypeMode=int8
  Product : Product  RndMeth=Zero
  Subtract : Sum  Inputs=+-  OutScaling=2^-10
  Subtract1 : Sum  OutScaling=2^-10
  Subtract2 : Sum  Inputs=+-  OutScaling=2^-10
  Subtract3 : Sum  OutScaling=2^-10
  tau_values : Outport  PortDimensions=4  OutputWhenDisabled=reset  InitialOutput=[0.0 0.0 0.0 0.0]
  wires:
  Mux2/1 -> tau_values/1
  Divide/1 -> Data Store Write3/1, Divide2/1
  Add/1 -> Divide/2
  Data Store Read3/1 -> Add/2, Mux2/1
  Constant2/1 -> Divide/1
  Constant4/1 -> Add/1, Divide2/3
  Constant3/1 -> Data Store Write2/1, Mux2/2
  Divide1/1 -> Data Store Write4/1, Subtract/1
  M_GR1/1 -> Divide1/2
  Add1/1 -> Divide1/1
  M_GR/1 -> Add1/1
  Divide2/1 -> Add1/2
  Constant5/1 -> Divide2/2
  Phase 2/1 -> Data Store Write/1
  Gain/1 -> Subtract2/1
  Subtract/1 -> Subtract2/2, Subtract1/1
  Data Store Read1/1 -> Subtract/2, Divide3/1, Subtract3/1
  Constant/1 -> Math Function/2
  Subtract2/1 -> Product/1
  Product/1 -> Subtract1/2
  Subtract1/1 -> Data Store Write6/1, Mux2/3, Display/1
  Math Function/1 -> Product/2
  Divide3/1 -> Math Function/1
  Subtract3/1 -> Data Store Write5/1
  Constant1/1 -> Subtract3/2
  Constant6/1 -> Divide3/2
  MF_S/1 -> Gain/1
  Data Store Read4/1 -> Mux2/4

== system saturn_ib_stack/Saturn_IB_Stack/Saturn Instrument Unit (IU)/LVDA / LVDC/LVDC Iterative Guidance Mode/Improved Estimate of Total time-to-go ==
  note: Eqn. 4.4.48
  note: Eqn. 4.4.49
  note: Eqn. 4.4.50
  note: Convert vector to scalar magnitude:
      | not explicit in the EDD
  T_3_i_sec : Inport  Port=1  LatchInput=off
  tau_3_sec : Inport  Port=2  LatchInput=off
  Delta_V_prime_V : Inport  Port=3  LatchInput=off
  L_prime_y : Inport  Port=4  LatchInput=off
  L_prime_3 : Inport  Port=5  LatchInput=off
  Add10 : Sum  Inputs=+-  OutScaling=2^-10
  Add11 : Sum  OutScaling=2^-10
  Add12 : Sum  Inputs=+-  OutScaling=2^-10
  Divide2 : Product  Inputs=*/  OutScaling=2^-10
  Gain1 : Gain  Gain=0.5
  Gain5 : Gain  Gain=1/V_ex3_mps
  Math Function : Math  Operator=square  SaturateOnIntegerOverflow=on
  Product13 : Product  RndMeth=Zero
  Sum of Elements : Sum  Inputs=+  OutScaling=2^-10
  Delta_T_prime_3 : Outport
  L_3 : Outport  Port=2
  Delta_L_3 : Outport  Port=3
  wires:
  Math Function/1 -> Sum of Elements/1
  Divide2/1 -> Add10/1
  L_prime_y/1 -> Divide2/2, Add10/2
  Add10/1 -> Gain1/1
  Gain1/1 -> Add11/2, Product13/2, Delta_L_3/1
  L_prime_3/1 -> Add11/1
  Add12/1 -> Gain5/1
  Gain5/1 -> Product13/1
  tau_3_sec/1 -> Add12/1
  T_3_i_sec/1 -> Add12/2
  Product13/1 -> Delta_T_prime_3/1
  Delta_V_prime_V/1 -> Math Function/1
  Add11/1 -> L_3/1
  Sum of Elements/1 -> Divide2/1

== system saturn_ib_stack/Saturn_IB_Stack/Saturn Instrument Unit (IU)/LVDA / LVDC/LVDC Iterative Guidance Mode/M4V Transform ==
  phi_T_rad : Inport  Port=1  LatchInput=off
  11 : Fcn  Expr=u(2)
  {12,21,23,32} (4 alike) : Fcn  Expr=0.0
  13 : Fcn  Expr=u(1)
  22 : Fcn  Expr=1.0
  31 : Fcn  Expr=-u(1)
  33 : Fcn  Expr=u(2)
  Mux : Mux  Inputs=2
  Mux2 : Mux  Inputs=9
  Reshape 9x1->3x3 : simulink/Math Operations/Reshape  OutputDimensionality=Customize  OutputDimensions=[3,3]
  SinCos : aerolibutil/SinCos
  DCM : Outport  InitialOutput=0
  wires:
  33/1 -> Mux2/9
  23/1 -> Mux2/8
  13/1 -> Mux2/7
  32/1 -> Mux2/6
  22/1 -> Mux2/5
  12/1 -> Mux2/4
  31/1 -> Mux2/3
  21/1 -> Mux2/2
  11/1 -> Mux2/1
  Mux2/1 -> Reshape 9x1->3x3/1
  Reshape 9x1->3x3/1 -> DCM/1
  SinCos/1 -> Mux/1
  SinCos/2 -> Mux/2
  phi_T_rad/1 -> SinCos/1
  Mux/1 -> 22/1, 11/1, 21/1, 31/1, 12/1, 32/1, 13/1, 23/1, 33/1

== system saturn_ib_stack/Saturn_IB_Stack/Saturn Instrument Unit (IU)/LVDA / LVDC/LVDC Iterative Guidance Mode/MS4 Transform Matrix ==
  note: "MS4" matrix from LVDC
      | Equation Defining Document
      | page I-14-4
  A_z_deg : Inport  Port=1  LatchInput=off
  phi_L_deg : Inport  Port=2  LatchInput=off
  lambda_deg : Inport  Port=3  LatchInput=off
  i_deg : Inport  Port=4  LatchInput=off
  Angle Conversion1 : aerolibconvert/Angle Conversion  IU=deg  OU=rad
  Angle Conversion2 : aerolibconvert/Angle Conversion  IU=deg  OU=rad
  Mux : Mux  Inputs=3
  S-Frame to 4-Frame (MS4 matrix) : Subsystem  AncestorBlock="aerolibtransform2/Euler Angles to  Direction Cosine Matrix"
      mask Type: Euler2DCM
      mask Description: Determine the 3-by-3 direction cosine matrix (DCM) from launch and inclination parameters. The output DCM transform represents the MS4 matrix.
      mask Display: disp('MS4')
  DCM_0 : Outport  SampleTime=1.6
  wires:
  phi_L_deg/1 -> Mux/2
  lambda_deg/1 -> Mux/3
  A_z_deg/1 -> Mux/1
  Mux/1 -> Angle Conversion2/1
  S-Frame to 4-Frame (MS4 matrix)/1(DCM) -> DCM_0/1
  Angle Conversion2/1 -> S-Frame to 4-Frame (MS4 matrix)/1(Az phi_L lambda)
  i_deg/1 -> Angle Conversion1/1
  Angle Conversion1/1 -> S-Frame to 4-Frame (MS4 matrix)/2(i_rad)
